simulink model "LR_Traject_Sim_too_new"  (R2018b)
settings: Solver=ode4  StartTime=0  StopTime=300  FixedStep=0.05  RelTol=1e-7
model workspace (MAT data in the model file):
  Object = Simulink.LookupTable
  Object.Table = Simulink.lookuptable.Table
  Object.Table.Dimensions = [0 0]
  Object.Table.DataType = 'auto'
  Object.Table.FieldName = 'Table'
  Object.Breakpoints = Simulink.lookuptable.Breakpoint
  Object.Breakpoints.TunableSizeName = 'N1'
  Object.Breakpoints.Dimensions = [0 0]
  Object.Breakpoints.DataType = 'auto'
  Object.Breakpoints.FieldName = 'BP1'
  Object.SupportTunableSize = 0
  Object.StructTypeInfo = Simulink.lookuptable.StructTypeInfo
  Object.StructTypeInfo.DataScope = 'Auto'
undefined symbols (not defined in the file or in its folder): Conditions, Eng, Recovery, Roc
libraries: simulink_extras x1
settings Model: Creator=adamb  LastModifiedBy=Daniel
settings SolverCC: ZeroCrossAlgorithm=Adaptive
settings DataIOCC: SaveFormat=StructureWithTime
settings OptimizationCC: LifeSpan=inf
settings DebuggingCC: AlgebraicLoopMsg=none  ArtificialAlgebraicLoopMsg=none  SFExecutionAtInitializationDiag=none
settings HardwareCC: ProdBitPerSizeT=32  ProdBitPerPtrDiffT=32  ProdWordSize=32  ProdHWDeviceType=Specified
settings SFSimCC: SimUseLocalCustomCode=off
settings RTWCC: RTWUseLocalCustomCode=off
settings CodeAppCC: StateflowObjectComments=on
settings SimscapeCC: SimscapeNormalizeSystem=off
settings ConfigurationSet: Description=SimMechanics 2G

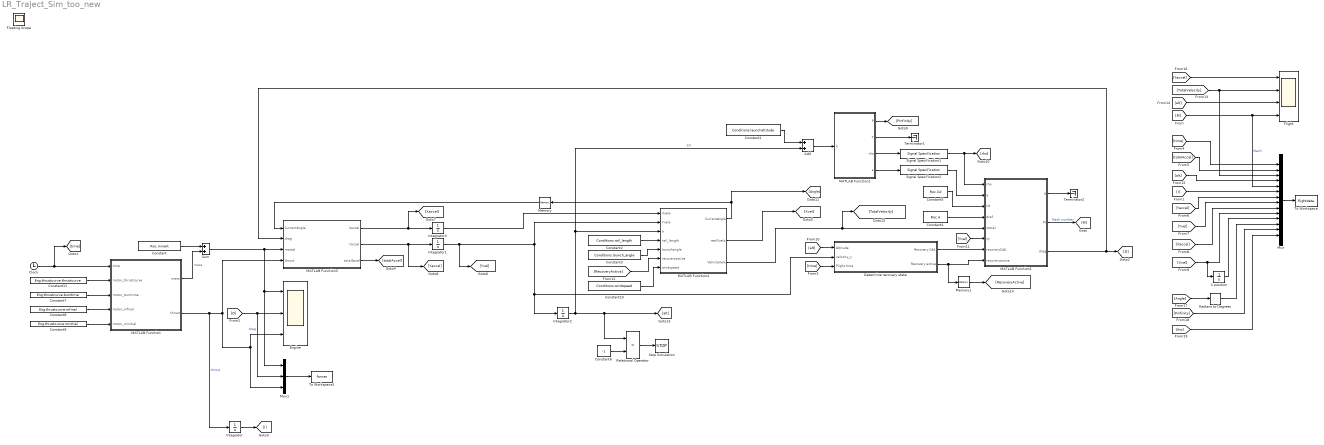
== system LR_Traject_Sim_too_new ==
  Add : Sum
  Clock : Clock
  Constant : Constant  Value=Roc.minert
  Constant1 : Constant  Value=Conditions.launchaltitude
  Constant10 : Constant  Value=Conditions.windspeed
  Constant11 : Constant  Value=Eng.thrustcurve.thrustcurve
  Constant2 : Constant  Value=Conditions.rail_length
  Constant3 : Constant  Value=Conditions.launch_angle
  Constant4 : Constant  Value=Roc.A
  Constant5 : Constant  Value=Roc.Cd  VectorParams1D=off
  Constant6 : Constant  Value=-1
  Constant7 : Constant  Value=Eng.thrustcurve.burntime
  Constant8 : Constant  Value=Eng.thrustcurve.mfinal
  Constant9 : Constant  Value=Eng.thrustcurve.minitial
  Determine recovery state : Subsystem
  Engine : Scope  NumInputPorts=3
  Flight : Scope  NumInputPorts=4
  Integrator{,1..3} (4 alike) : Integrator
  MATLAB Function : MATLAB Function  TreatAsAtomicUnit=on
  MATLAB Function1 : MATLAB Function  TreatAsAtomicUnit=on
  MATLAB Function2 : MATLAB Function  TreatAsAtomicUnit=on
  MATLAB Function3 : MATLAB Function  TreatAsAtomicUnit=on
  MATLAB Function4 : MATLAB Function  TreatAsAtomicUnit=on
  Memory : Memory
  Memory1 : Memory
  Mux : Mux  Inputs=14
  Mux1 : Mux  Inputs=3
  Radians to Degrees : simulink_extras/Transformations/Radians to Degrees
  Relational Operator : RelationalOperator  Operator=<  OutDataTypeStr=boolean  RndMeth=Nearest
  Signal Specification1 : SignalSpecification  OutDataTypeStr=double  Dimensions=1
  Signal Specification2 : SignalSpecification  OutDataTypeStr=double  Dimensions=1
  Stop Simulation : Stop
  Sum : Sum
  Terminator1 : Terminator
  Terminator2 : Terminator
  To Workspace : ToWorkspace  VariableName=flightdata  SampleTime=-1
  To Workspace1 : ToWorkspace  VariableName=forces  SampleTime=-1
  X position : Integrator
  Floating Scope : Scope
  wires:
  MATLAB Function/2(thrust) -> Integrator/1, Mux1/3, Engine/3, MATLAB Function3/4(thrust)  "thrust"
  Integrator1/1 -> [Yvel], Integrator2/1, Determine recovery state/2(velocity_y), MATLAB Function4/2(Yvelo)
  Integrator2/1 -> [alt], Relational Operator/1, Add/2, MATLAB Function4/3(h)  "alt"
  Constant4/1 -> MATLAB Function1/4(Aref)
  Constant5/1 -> MATLAB Function1/3(Cd)
  MATLAB Function1/2(M) -> [M]  "Mach number"
  [M] -> Mux/5, Flight/4  "Mach"
  Relational Operator/1 -> Stop Simulation/1
  Constant6/1 -> Relational Operator/2
  Mux/1 -> To Workspace/1
  MATLAB Function2/2(T) -> Terminator1/1
  [D] -> Mux1/2, Engine/2  "drag"
  Mux1/1 -> To Workspace1/1
  MATLAB Function1/1(q) -> Terminator2/1
  MATLAB Function2/1(P) -> [Pinfinity]
  Clock/1 -> MATLAB Function/1(time), [time]
  [time] -> Mux/1
  MATLAB Function3/2(Yaccel) -> Integrator1/1, [Yaccel]
  Integrator3/1 -> MATLAB Function4/1(Xvelo)
  MATLAB Function4/3(VehicleVelo) -> [TotalVelocity], MATLAB Function1/5(vtotal)
  Integrator/1 -> [I]
  [I] -> Mux/6
  Add/1 -> MATLAB Function2/1(h)
  Constant1/1 -> Add/1
  MATLAB Function4/1(CurrentAngle) -> Memory/1, [Angle]
  Constant2/1 -> MATLAB Function4/4(rail_length)
  Constant3/1 -> MATLAB Function4/5(launchangle)
  [totalAccel] -> Mux/2
  [Xaccel] -> Mux/9
  [Xvel] -> Mux/10, X position/1
  [Yvel] -> Mux/8
  [Yaccel] -> Mux/7
  X position/1 -> Mux/11
  MATLAB Function3/1(Xaccel) -> Integrator3/1, [Xaccel]
  MATLAB Function3/3(totalAccel) -> [totalAccel]
  Constant/1 -> Sum/1
  Sum/1 -> Mux1/1, Engine/1, MATLAB Function3/3(mtotal)
  Constant11/1 -> MATLAB Function/2(motor_thrustcurve)
  Constant7/1 -> MATLAB Function/3(motor_burntime)
  Constant8/1 -> MATLAB Function/4(motor_mfinal)
  Constant9/1 -> MATLAB Function/5(motor_minitial)
  [time] -> Determine recovery state/3(Flight time)
  [alt] -> Determine recovery state/1(Altitude)
  MATLAB Function/1(mass) -> Sum/2  "mass"
  Signal Specification1/1 -> [rho], MATLAB Function1/1(rho)
  Signal Specification2/1 -> MATLAB Function1/2(a)
  MATLAB Function2/4(a) -> Signal Specification2/1
  MATLAB Function2/3(rho) -> Signal Specification1/1
  Determine recovery state/1(Recovery CdA) -> MATLAB Function1/7(recoveryCdA)
  Memory/1 -> MATLAB Function3/1(CurrentAngle)
  Determine recovery state/2(Recovery active) -> Memory1/1, MATLAB Function1/8(recoveryactive)
  [Yvel] -> MATLAB Function1/6(vy)
  Memory1/1 -> [RecoveryActive]
  [RecoveryActive] -> MATLAB Function4/6(recoveryactive)
  [TotalVelocity] -> Flight/2, Mux/3
  [alt] -> Flight/3
  [alt] -> Mux/4
  [Yaccel] -> Flight/1
  [Pinfinity] -> Mux/13
  [rho] -> Mux/14
  [Angle] -> Radians to Degrees/1
  Radians to Degrees/1 -> Mux/12
  MATLAB Function4/2(realXvelo) -> [Xvel]
  Constant10/1 -> MATLAB Function4/7(windspeed)
  MATLAB Function1/3(drag) -> MATLAB Function3/2(drag), [D]

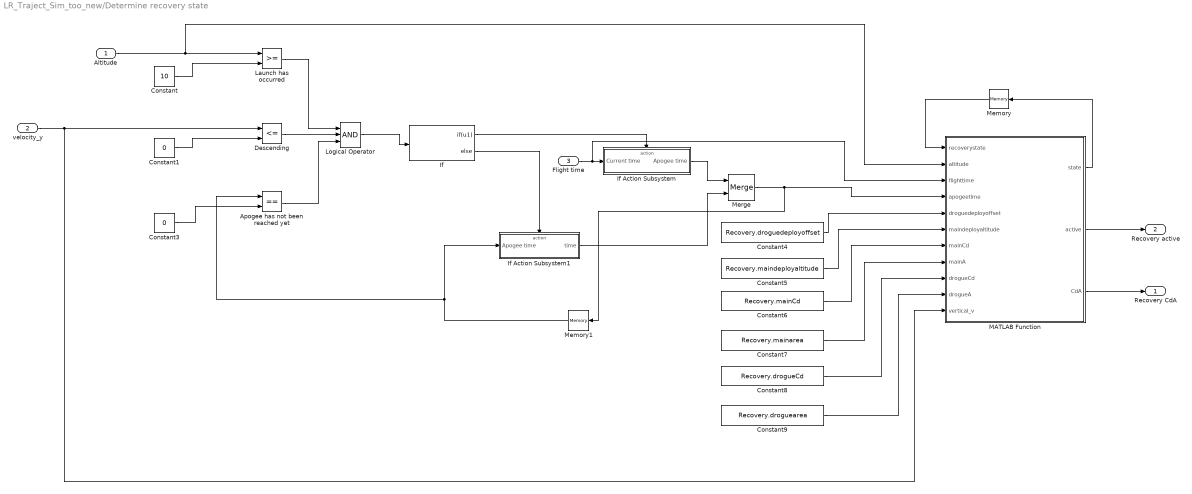
== system LR_Traject_Sim_too_new/Determine recovery state ==
  Altitude : Inport
  velocity_y : Inport  Port=2
  Flight time : Inport  Port=3
  Apogee has not been reached yet : RelationalOperator  Operator===  OutDataTypeStr=boolean  RndMeth=Simplest
  Constant : Constant  Value=10
  Constant1 : Constant  Value=0
  Constant3 : Constant  Value=0
  Constant4 : Constant  Value=Recovery.droguedeployoffset
  Constant5 : Constant  Value=Recovery.maindeployaltitude
  Constant6 : Constant  Value=Recovery.mainCd
  Constant7 : Constant  Value=Recovery.mainarea
  Constant8 : Constant  Value=Recovery.drogueCd
  Constant9 : Constant  Value=Recovery.droguearea
  Descending : RelationalOperator  Operator=<=  OutDataTypeStr=boolean  RndMeth=Simplest
  If : If  IfExpression=u1
  If Action Subsystem : Subsystem  TreatAsAtomicUnit=on
  If Action Subsystem1 : Subsystem  TreatAsAtomicUnit=on
  Launch has occurred : RelationalOperator  OutDataTypeStr=boolean  RndMeth=Simplest
  Logical Operator : Logic  Inputs=3  AllPortsSameDT=off  OutDataTypeStr=boolean
  MATLAB Function : MATLAB Function  TreatAsAtomicUnit=on
  Memory : Memory
  Memory1 : Memory
  Merge : Merge
  Recovery CdA : Outport  OutDataTypeStr=double  PortDimensions=1
  Recovery active : Outport  Port=2  OutDataTypeStr=uint8  PortDimensions=1
  wires:
  Altitude/1 -> MATLAB Function/2(altitude), Launch has occurred/1
  Constant/1 -> Launch has occurred/2
  velocity_y/1 -> Descending/1, MATLAB Function/11(vertical_v)
  Constant1/1 -> Descending/2
  Launch has occurred/1 -> Logical Operator/1
  Descending/1 -> Logical Operator/2
  Constant3/1 -> Apogee has not been reached yet/2
  Memory1/1 -> Apogee has not been reached yet/1, If Action Subsystem1/1(Apogee time)
  Apogee has not been reached yet/1 -> Logical Operator/3
  Logical Operator/1 -> If/1
  If/1 -> If Action Subsystem/Action
  If/2 -> If Action Subsystem1/Action
  If Action Subsystem/1(Apogee time) -> Merge/1
  If Action Subsystem1/1(time) -> Merge/2
  Merge/1 -> Memory1/1, MATLAB Function/4(apogeetime)
  Constant4/1 -> MATLAB Function/5(droguedeployoffset)
  Constant5/1 -> MATLAB Function/6(maindeployaltitude)
  MATLAB Function/2(active) -> Recovery active/1
  MATLAB Function/3(CdA) -> Recovery CdA/1
  MATLAB Function/1(state) -> Memory/1
  Memory/1 -> MATLAB Function/1(recoverystate)
  Flight time/1 -> MATLAB Function/3(flighttime), If Action Subsystem/1(Current time)
  Constant6/1 -> MATLAB Function/7(mainCd)
  Constant8/1 -> MATLAB Function/9(drogueCd)
  Constant9/1 -> MATLAB Function/10(drogueA)
  Constant7/1 -> MATLAB Function/8(mainA)

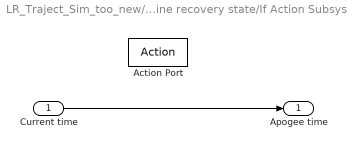
== system LR_Traject_Sim_too_new/Determine recovery state/If Action Subsystem ==
  Current time : Inport
  Action Port : ActionPort  ActionType=then
  Apogee time : Outport
  wires:
  Current time/1 -> Apogee time/1

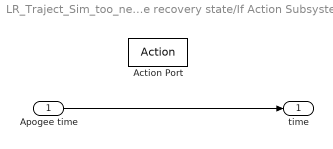
== system LR_Traject_Sim_too_new/Determine recovery state/If Action Subsystem1 ==
  Apogee time : Inport
  Action Port : ActionPort  ActionType=else
  time : Outport
  wires:
  Apogee time/1 -> time/1

== matlab function LR_Traject_Sim_too_new/MATLAB Function1 ==
  data: rho input; a input; q output; M output; Cd input; Aref input; vtotal input; drag output; vy input; recoveryCdA input; recoveryactive input
function [q,M,drag] = AeroComputation(rho,a,Cd,Aref,vtotal, vy, recoveryCdA, recoveryactive)

M = abs(vtotal/a); % Mach #

if recoveryactive == 0
    v = vtotal;
else
    %fprintf('vtotal = %f, vx = %f\n', vtotal, vx);
    v = vy;
end

q = 0.5 * rho * v.^2 * sign(v); % qbar, Dynamic Pressure
    
A = Aref(1);
CdM = interp1(Cd(1,:),Cd(2,:),M); % Interpolates the Cd based on M

if ~recoveryactive
    drag = q*A*CdM;
else
    drag = q * recoveryCdA;
end

%fprintf('Velocity is %f, drag is %f, rho is %f, a is %f, Cdm is %f\n', v, drag, rho, a, CdM);


end

== matlab function LR_Traject_Sim_too_new/Determine recovery state/MATLAB Function ==
  data: state output uint8; recoverystate input; altitude input; flighttime input; active output uint8 size=1; apogeetime input; droguedeployoffset input; maindeployaltitude input; mainCd input; mainA input; drogueCd input; drogueA input; vertical_v input; CdA output
function [state, active, CdA] = determineCdA(recoverystate, altitude,...
    flighttime, apogeetime, droguedeployoffset, maindeployaltitude,...
    mainCd, mainA, drogueCd, drogueA, vertical_v)
state = recoverystate; %Match previous by default, change if required
CdA = 0;
%This is all needlessly complicated to make it easy to implement a more
%complex recovery system performance calculation later - time/altitude
%since deployment could easily be passed through to the chute performance
%functions as well, or whatever other parameters are needed
if apogeetime > 0 && apogeetime + droguedeployoffset <= flighttime && recoverystate == 0
    state = uint8(1); %Drogue deployed
elseif recoverystate == 1 && altitude < maindeployaltitude
    state = uint8(2);
end
if state == 1
    CdA = droguechuteperformance(drogueCd, drogueA);
elseif state == 2
    CdA = mainchuteperformance(mainCd, mainA);
end

if recoverystate
    active = uint8(1);
else
    active = uint8(0);
end

end

== matlab function LR_Traject_Sim_too_new/MATLAB Function2 ==
  data: h input; P output; T output; rho output; a output
function [P,T,rho,a] = AtmosParams(h)

[P,rho,T,a] = StdAtmos(h);

end

== matlab function LR_Traject_Sim_too_new/MATLAB Function3 ==
  data: CurrentAngle input; drag input; mtotal input; Xaccel output; thrust input; Yaccel output; totalAccel output
function [Xaccel, Yaccel, totalAccel] = AccelerationComponents(CurrentAngle, drag, mtotal, thrust)

%Direction of current velocity vector equals Current Angle
%Thrust and drag are assumed along the axis of the velocity
%Gravity is constant 9.81m/s^2 along the y-axis

%Constants
AccelGravity = -9.81;

AccelDrag = drag/mtotal; %Acceleration caused by drag
AccelThrust = thrust/mtotal; %Acceleration caused by Thrust
AccelRocket = AccelThrust-AccelDrag; %Acceleration of Rocket
Yaccel = AccelRocket * cos(CurrentAngle) + AccelGravity; %Acceleration of Rocket in Y Direction
Xaccel = AccelRocket * sin(CurrentAngle); %Acceleration of rocket in x direction
totalAccel = sqrt(Xaccel^2 + Yaccel^2);

== matlab function LR_Traject_Sim_too_new/MATLAB Function4 ==
  data: Xvelo input; CurrentAngle output; realXvelo output; Yvelo input; h input; rail_length input; VehicleVelo output; launchangle input; recoveryactive input; windspeed input
function [CurrentAngle, realXvelo, VehicleVelo]  = CurrentAngle(Xvelo,Yvelo, h, rail_length, launchangle, recoveryactive, windspeed)

%This function's main purpose is to calculate current vehicle angle without
%using two simulink math blocks vs one function block.

%Pretty cool huh?

CurrentAngle = atan(Xvelo / Yvelo);
VehicleVelo = sqrt(Xvelo.^2 + Yvelo.^2);
realXvelo = Xvelo;

if h < rail_length
    CurrentAngle = launchangle;
end

if recoveryactive
    CurrentAngle = 0;
    realXvelo = -1 * windspeed;
end
end

== matlab function LR_Traject_Sim_too_new/MATLAB Function ==
  data: mass output; time input; thrust output; motor_thrustcurve input; motor_burntime input; motor_mfinal input; motor_minitial input
function [mass, thrust] = solidThrust(time, motor_thrustcurve, motor_burntime, motor_mfinal, motor_minitial)

data = motor_thrustcurve;
% If t is after the end of the data, thrust is 0
if time >= data(end, 1)
    thrust = 0;
else

    % Find the data point before this time
    for before = 1:(length(data) - 1)
        if data(before + 1, 1) > time
            break;
        end
    end
    % And the data point after this time
    after = before + 1;
    % Calculate thrust through linear interpolation between the thrust before
    % and the thrust after the target time
    thrust = data(before, 2) + (time - data(before, 1)) * ...
        (data(after, 2) - data(before, 2)) / ...
        (data(after, 1) - data(before, 1));
end

if time >= motor_burntime
    mass = motor_mfinal;
else
    mass = motor_minitial - (time / motor_burntime) * (motor_minitial - motor_mfinal);
end
end
